simulink model "SS_XRay_sim"  (R2025a)
settings: Solver=VariableStepAuto  StartTime=0.0  StopTime=10.0  RelTol=1e-3
settings Model: Creator=Admin  LastModifiedBy=Admin

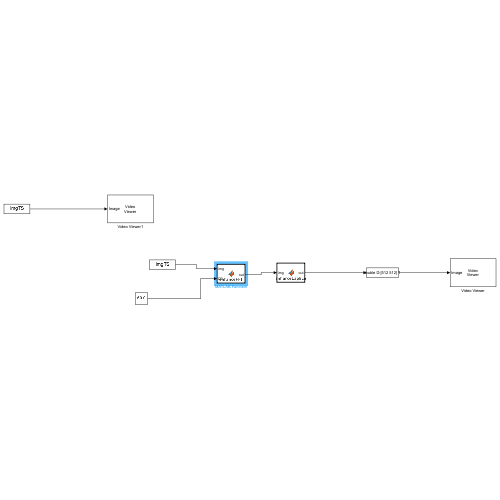
[thumbnail: Simulink's stored preview of the top-level diagram]
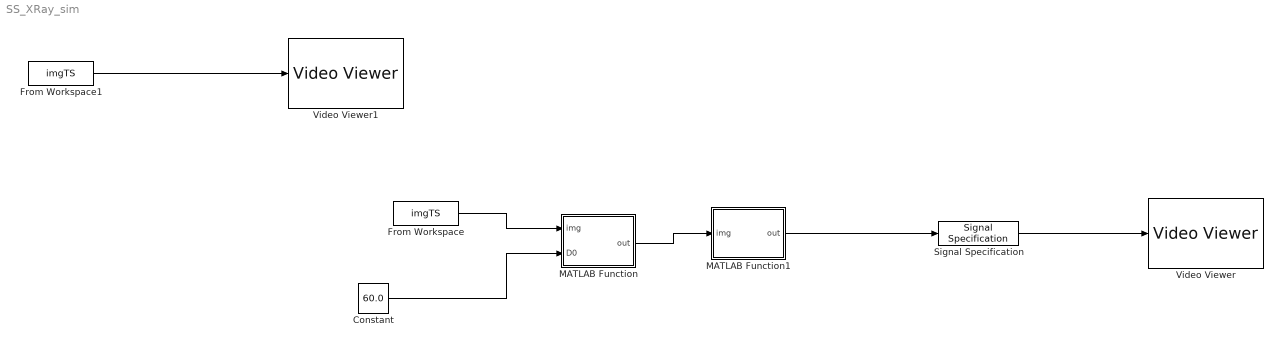
== system SS_XRay_sim ==
  Constant : Constant  Value=60.0  OutDataTypeStr=double  SampleTime=1
  From Workspace : FromWorkspace  VariableName=imgTS  SampleTime=1
  From Workspace1 : FromWorkspace  VariableName=imgTS  SampleTime=1
  MATLAB Function : MATLAB Function  TreatAsAtomicUnit=on
  MATLAB Function1 : MATLAB Function  TreatAsAtomicUnit=on
  Signal Specification : SignalSpecification  OutDataTypeStr=double  Dimensions=[512 512]  SampleTime=1
  Video Viewer : VideoViewer  FigPos=[1 718 1366 621]
  Video Viewer1 : VideoViewer  FigPos=[1 718 1366 621]
  wires:
  Signal Specification/1 -> Video Viewer/1
  Constant/1 -> MATLAB Function/2(D0)
  From Workspace/1 -> MATLAB Function/1(img)
  MATLAB Function/1(out) -> MATLAB Function1/1(img)
  MATLAB Function1/1(out) -> Signal Specification/1
  From Workspace1/1 -> Video Viewer1/1

== matlab function SS_XRay_sim/MATLAB Function ==
  data: img input; out output; D0 input
function out = enhanceFFT(img, D0)

img = im2double(img);
orig = imresize(img, [512 512]);

% FFT
F = fftshift(fft2(orig));
[rows, cols] = size(orig);
[u,v] = meshgrid(-floor(cols/2):ceil(cols/2)-1, -floor(rows/2):ceil(rows/2)-1);
D = sqrt(u.^2 + v.^2);

% Filters
LP = exp(-(D.^2)/(2*(D0^2)));
HP = 1 - LP;

% Extract detail
detail = real(ifft2(ifftshift(F .* HP)));

% ADD THE DETAIL BACK (THE KEY FIX)
alpha = 0.3;      % strength of sharpening (you can adjust 0.3–0.8)
out = orig + alpha * detail;

% FINAL normalize (important but mild)
out = out - min(out(:));
out = out ./ (max(out(:)) + eps);

end

== matlab function SS_XRay_sim/MATLAB Function1 ==
  data: img input; out output
function out = enhanceLaplace(img)
%#codegen

% Laplacian operator (Laplace transform concept)
L = del2(img);  % second derivative

alpha = 0.4;  % sharpening strength

out = img + alpha * L;

% normalize
out = out - min(out(:));
out = out ./ (max(out(:)) + eps);

end
